simulink subsystem "trajectory_generation_ref_subsys_cont"  (R2023b)
settings: Solver=VariableStepAuto  StartTime=0.0  StopTime=10.0  RelTol=1e-3
values from neighbouring files (symbols this model uses):
  H_0_init = [7.85046229342e-17 1 0 0 1 -7.85046229342e-17 0 0 0 0 -1 0 ... (16 elements, 4x4)]    [matlab.mat]    (also in parameters.m = hom_transform_endeffector(q_0, param_robot))
  param_traj_allg =     [matlab.mat]
  xe0 = [0.392090710168 0.392090710168 0.5211 0 0.707106781187 0.707106781187 0]    [matlab.mat]    (also in parameters.m = temp)
  xeT = [0.392090710168 0.392090710168 0.5211 0 0.382683432365 0.923879532511 0]    [matlab.mat]    (also in parameters.m = xe0)
settings Model: Creator=emu  LastModifiedBy=emu

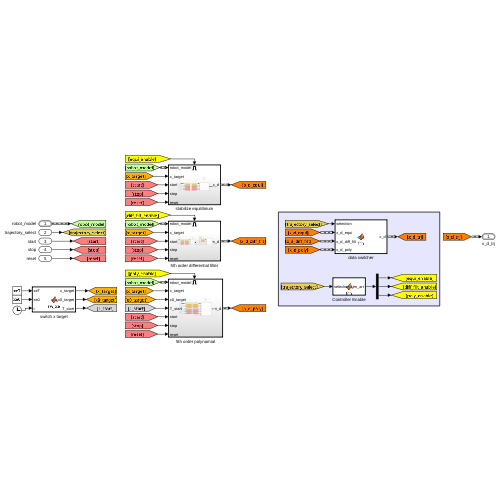
[thumbnail: Simulink's stored preview of the top-level diagram]
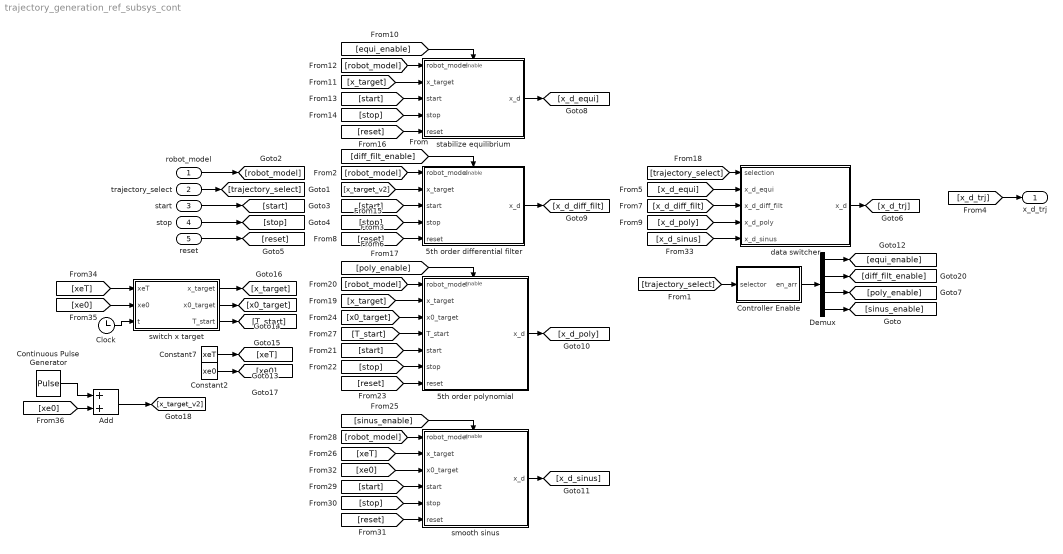
== system trajectory_generation_ref_subsys_cont ==
  robot_model : Inport  OutDataTypeStr=Bus: robot_model
  trajectory_select : Inport  Port=2
  start : Inport  Port=3
  stop : Inport  Port=4
  reset : Inport  Port=5
  5th order differential filter : Subsystem
  5th order polynomial : Subsystem
  Add : Sum
  Clock : Clock
  Constant2 : Constant  Value=xe0
  Constant7 : Constant  Value=xeT
  Continuous Pulse Generator : DiscretePulseGenerator  PulseType=Time based  Amplitude=xeT-xe0  Period=param_traj_allg.T_switch*2  PulseWidth=50
  Controller Enable : MATLAB Function  TreatAsAtomicUnit=on
  Demux : Demux
  data switcher : MATLAB Function  TreatAsAtomicUnit=on
  smooth sinus : Subsystem
  stabilize equilibrium : Subsystem
  switch x target : MATLAB Function  TreatAsAtomicUnit=on
  x_d_trj : Outport  OutDataTypeStr=Bus: x_d
  wires:
  [reset] -> 5th order differential filter/5(reset)
  [x_d_equi] -> data switcher/2(x_d_equi)
  [poly_enable] -> 5th order polynomial/Enable
  [x_target] -> stabilize equilibrium/2(x_target)
  [robot_model] -> 5th order differential filter/1(robot_model)
  Clock/1 -> switch x target/3(t)
  [xe0] -> switch x target/2(xe0)
  stop/1 -> [stop]
  Demux/2 -> [diff_filt_enable]
  switch x target/2(x0_target) -> [x0_target]
  start/1 -> [start]
  Demux/3 -> [poly_enable]
  [diff_filt_enable] -> 5th order differential filter/Enable
  [reset] -> stabilize equilibrium/5(reset)
  reset/1 -> [reset]
  [stop] -> 5th order polynomial/6(stop)
  5th order polynomial/1(x_d) -> [x_d_poly]
  [stop] -> 5th order differential filter/4(stop)
  [x_d_poly] -> data switcher/4(x_d_poly)
  data switcher/1(x_d) -> [x_d_trj]
  [T_start] -> 5th order polynomial/4(T_start)
  [x_d_trj] -> x_d_trj/1
  [x_target_v2] -> 5th order differential filter/2(x_target)
  [x_target] -> 5th order polynomial/2(x_target)
  switch x target/3(T_start) -> [T_start]
  [robot_model] -> 5th order polynomial/1(robot_model)
  robot_model/1 -> [robot_model]
  trajectory_select/1 -> [trajectory_select]
  [x0_target] -> 5th order polynomial/3(x0_target)
  [trajectory_select] -> Controller Enable/1(selector)
  [stop] -> stabilize equilibrium/4(stop)
  [start] -> stabilize equilibrium/3(start)
  stabilize equilibrium/1(x_d) -> [x_d_equi]
  5th order differential filter/1(x_d) -> [x_d_diff_filt]
  [robot_model] -> stabilize equilibrium/1(robot_model)
  [reset] -> 5th order polynomial/7(reset)
  [x_d_diff_filt] -> data switcher/3(x_d_diff_filt)
  switch x target/1(x_target) -> [x_target]
  Controller Enable/1(en_arr) -> Demux/1
  [start] -> 5th order polynomial/5(start)
  [xeT] -> switch x target/1(xeT)
  [equi_enable] -> stabilize equilibrium/Enable
  Demux/1 -> [equi_enable]
  [trajectory_select] -> data switcher/1(selection)
  [start] -> 5th order differential filter/3(start)
  [start] -> smooth sinus/4(start)
  [reset] -> smooth sinus/6(reset)
  [xe0] -> smooth sinus/3(x0_target)
  [robot_model] -> smooth sinus/1(robot_model)
  [xeT] -> smooth sinus/2(x_target)
  smooth sinus/1(x_d) -> [x_d_sinus]
  [stop] -> smooth sinus/5(stop)
  [sinus_enable] -> smooth sinus/Enable
  Demux/4 -> [sinus_enable]
  [x_d_sinus] -> data switcher/5(x_d_sinus)
  Constant7/1 -> [xeT]
  Constant2/1 -> [xe0]
  Continuous Pulse Generator/1 -> Add/1
  [xe0] -> Add/2
  Add/1 -> [x_target_v2]

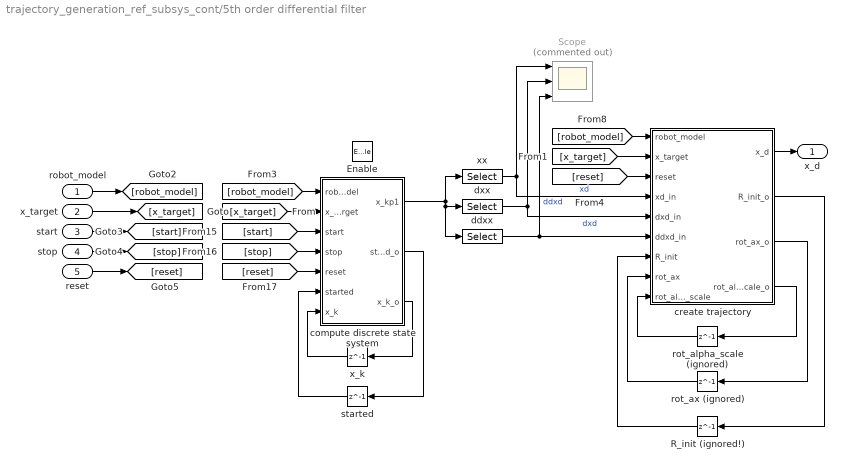
== system trajectory_generation_ref_subsys_cont/5th order differential filter ==
  robot_model : Inport
  x_target : Inport  Port=2
  start : Inport  Port=3
  stop : Inport  Port=4
  reset : Inport  Port=5
  Enable : EnablePort
  R_init (ignored!) : Delay  DelayLength=1  InitialCondition=eye(3)
  Scope : Scope  Commented=on  NumInputPorts=3
  compute discrete state system : MATLAB Function  TreatAsAtomicUnit=on
  create trajectory : MATLAB Function  TreatAsAtomicUnit=on
  ddxx : Selector  InputPortWidth=24  IndexOptions=Index vector (dialog)  Indices=selector_index3  OutputSizes=1
  dxx : Selector  InputPortWidth=24  IndexOptions=Index vector (dialog)  Indices=selector_index2  OutputSizes=1
  rot_alpha_scale (ignored) : Delay  DelayLength=1  InitialCondition=0
  rot_ax (ignored) : Delay  DelayLength=1  InitialCondition=[1;0;0]
  started : Delay  DelayLength=1
  x_k : Delay  DelayLength=1  InitialCondition=[reshape([H_0_init(1:3,4) zeros(3,5)]', 6*3,1)]
  xx : Selector  InputPortWidth=24  IndexOptions=Index vector (dialog)  Indices=selector_index1  OutputSizes=1
  x_d : Outport  OutDataTypeStr=Bus: x_d
  wires:
  R_init (ignored!)/1 -> create trajectory/7(R_init)
  rot_ax (ignored)/1 -> create trajectory/8(rot_ax)
  rot_alpha_scale (ignored)/1 -> create trajectory/9(rot_alpha_scale)
  create trajectory/2(R_init_o) -> R_init (ignored!)/1
  create trajectory/3(rot_ax_o) -> rot_ax (ignored)/1
  create trajectory/4(rot_alpha_scale_o) -> rot_alpha_scale (ignored)/1
  started/1 -> compute discrete state system/6(started)
  x_k/1 -> compute discrete state system/7(x_k)
  compute discrete state system/3(x_k_o) -> x_k/1
  compute discrete state system/2(started_o) -> started/1
  [x_target] -> compute discrete state system/2(x_target)
  [x_target] -> create trajectory/2(x_target)
  x_target/1 -> [x_target]
  ddxx/1 -> create trajectory/6(ddxd_in), Scope/3  "ddxd"
  [start] -> compute discrete state system/3(start)
  xx/1 -> Scope/1, create trajectory/4(xd_in)  "xd"
  [robot_model] -> compute discrete state system/1(robot_model)
  [stop] -> compute discrete state system/4(stop)
  create trajectory/1(x_d) -> x_d/1
  dxx/1 -> Scope/2, create trajectory/5(dxd_in)  "dxd"
  compute discrete state system/1(x_kp1) -> xx/1, dxx/1, ddxx/1
  [reset] -> compute discrete state system/5(reset)
  robot_model/1 -> [robot_model]
  start/1 -> [start]
  reset/1 -> [reset]
  [reset] -> create trajectory/3(reset)
  stop/1 -> [stop]
  [robot_model] -> create trajectory/1(robot_model)

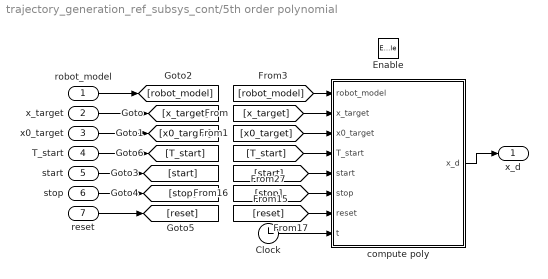
== system trajectory_generation_ref_subsys_cont/5th order polynomial ==
  robot_model : Inport
  x_target : Inport  Port=2
  x0_target : Inport  Port=3
  T_start : Inport  Port=4
  start : Inport  Port=5
  stop : Inport  Port=6
  reset : Inport  Port=7
  Enable : EnablePort
  Clock : Clock
  compute poly : MATLAB Function  TreatAsAtomicUnit=on
  x_d : Outport  OutDataTypeStr=Bus: x_d
  wires:
  [T_start] -> compute poly/4(T_start)
  T_start/1 -> [T_start]
  [x0_target] -> compute poly/3(x0_target)
  x0_target/1 -> [x0_target]
  Clock/1 -> compute poly/8(t)
  [start] -> compute poly/5(start)
  [stop] -> compute poly/6(stop)
  compute poly/1(x_d) -> x_d/1
  [reset] -> compute poly/7(reset)
  robot_model/1 -> [robot_model]
  start/1 -> [start]
  reset/1 -> [reset]
  stop/1 -> [stop]
  x_target/1 -> [x_target]
  [x_target] -> compute poly/2(x_target)
  [robot_model] -> compute poly/1(robot_model)

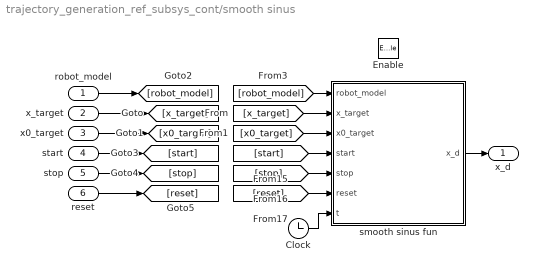
== system trajectory_generation_ref_subsys_cont/smooth sinus ==
  robot_model : Inport
  x_target : Inport  Port=2
  x0_target : Inport  Port=3
  start : Inport  Port=4
  stop : Inport  Port=5
  reset : Inport  Port=6
  Enable : EnablePort
  Clock : Clock
  smooth sinus fun : MATLAB Function  TreatAsAtomicUnit=on
  x_d : Outport  OutDataTypeStr=Bus: x_d
  wires:
  [robot_model] -> smooth sinus fun/1(robot_model)
  [x_target] -> smooth sinus fun/2(x_target)
  x_target/1 -> [x_target]
  stop/1 -> [stop]
  reset/1 -> [reset]
  start/1 -> [start]
  robot_model/1 -> [robot_model]
  [reset] -> smooth sinus fun/6(reset)
  smooth sinus fun/1(x_d) -> x_d/1
  [stop] -> smooth sinus fun/5(stop)
  [start] -> smooth sinus fun/4(start)
  Clock/1 -> smooth sinus fun/7(t)
  x0_target/1 -> [x0_target]
  [x0_target] -> smooth sinus fun/3(x0_target)

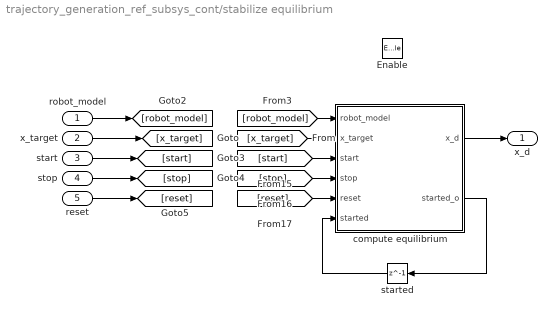
== system trajectory_generation_ref_subsys_cont/stabilize equilibrium ==
  robot_model : Inport
  x_target : Inport  Port=2
  start : Inport  Port=3
  stop : Inport  Port=4
  reset : Inport  Port=5
  Enable : EnablePort
  compute equilibrium : MATLAB Function  TreatAsAtomicUnit=on
  started : Delay  DelayLength=1
  x_d : Outport  OutDataTypeStr=Bus: x_d
  wires:
  compute equilibrium/2(started_o) -> started/1
  started/1 -> compute equilibrium/6(started)
  [robot_model] -> compute equilibrium/1(robot_model)
  [x_target] -> compute equilibrium/2(x_target)
  x_target/1 -> [x_target]
  stop/1 -> [stop]
  reset/1 -> [reset]
  start/1 -> [start]
  robot_model/1 -> [robot_model]
  [reset] -> compute equilibrium/5(reset)
  compute equilibrium/1(x_d) -> x_d/1
  [stop] -> compute equilibrium/4(stop)
  [start] -> compute equilibrium/3(start)

== matlab function trajectory_generation_ref_subsys_cont/switch x target ==
  data: x_target output; x0_target output; xeT input; xe0 input; t input; param_vis parameter; T_start output
function [x_target, x0_target, T_start]= sw_xe(xeT, xe0, t, param_vis)

if(t < param_vis.T/2)
    x_target = xeT;
    x0_target = xe0;
    flag = 0;
else
    x_target = xe0;
    x0_target = xeT;
    flag = 1;
end

if(flag == 0)
    T_start = 0;
else
    T_start = param_vis.T/2;
end

== matlab function trajectory_generation_ref_subsys_cont/smooth sinus/smooth sinus fun ==
  settings: sampleTime=param_global.Ta
  data: robot_model input Bus: robot_model; x_target input; x0_target input; start input; stop input; reset input; t input; x_d output Bus: x_d; param_traj_sin_poly parameter
function x_d  = ss_z(robot_model, x_target, x0_target, start, stop, reset, t, param_traj_sin_poly)

persistent started;

if(reset == 1 || isempty(started))
    started = false;
end

if(start == 1 && stop == 0 && ~started)
    started = true;
end

if(stop == 1)
    started = false;
end

if(started)
    T = param_traj_sin_poly.T;
    omega = param_traj_sin_poly.omega;
    phi = param_traj_sin_poly.phi;
    if(t > T)
        s =    1;
        s_p =  0;
        s_pp = 0;
    else
        [s, s_p, s_pp] = trajectory_poly(t, 0, 1, T);
    end
    xT = x_target(1);
    x0 = x0_target(1);

    a = (xT - x0)/2; % width of sinus movement

    sin_t = a*sin(omega*t - phi);
    cos_t = a*cos(omega*t - phi);

    %p_d = x0 + a*sin(omega*t)*s;
    %p_d_p = a*omega*cos(omega*t)*s + a*sin(omega*t)*s_p;
    %p_d_pp = -omega*a*sin(omega*t)*s + 2*omega*cos(omega*t)*s_p + a*sin(omega*t) * s_pp;
    x_ref = x0 + (a + sin_t) * s;
    x_ref_p =    cos_t * omega * s   + sin_t * s_p;
    x_ref_pp =  -sin_t * omega^2 * s + cos_t * s_p * omega * 2 + sin_t * s_pp;

    x_d.p_d = [x_ref; x_target(2:3)];
    x_d.p_d_p = [x_ref_p; x_target(2:3)];
    x_d.p_d_pp = [x_ref_pp; x_target(2:3)];
    
    x_d.q_d = zeros(4,1);
    x_d.omega_d   = zeros(3,1);
    x_d.omega_d_p = zeros(3,1);
else
    H = robot_model.H;
    p_e = H(1:3, 4);

    x_d.p_d = p_e;
    x_d.p_d_p =  zeros(3,1);
    x_d.p_d_pp = zeros(3,1);
    x_d.q_d = zeros(4,1);
    x_d.omega_d   = zeros(3,1);
    x_d.omega_d_p = zeros(3,1);
end

== matlab function trajectory_generation_ref_subsys_cont/5th order differential filter/compute discrete state system ==
  settings: sampleTime=param_global.Ta
  data: robot_model input Bus: robot_model; x_target input; start input; stop input; reset input; started input; x_k input; x_kp1 output; param_traj_filter parameter; started_o output; x_k_o output
function [x_kp1, started_o, x_k_o]  = ss_z(robot_model, x_target, start, stop, reset, started, x_k, param_traj_filter)

if(reset == 1)
    H = robot_model.H;
    yt_init = H(1:3, 4);
    %x_target = eval_path_t(theta, 1, path_param);
    %x;d/dt x;d^2/dt^2 x; y;d/dt y;d^2/dt^2 y; z;d/dt z;d^2/dt^2 z; alpha;d/dt alpha;d^2/dt^2 alpha
    x_0 = [yt_init(1);0;0;0;0;0; yt_init(2);0;0;0;0;0; yt_init(3);0;0;0;0;0; 0;0;0;0;0;0];
    x_k = x_0;
    started = false;
end

if(start == 1 && stop == 0 && ~started)
    started = true;
end

if(stop == 1)
    started = false;
end

if(started)
    Phi = param_traj_filter.Phi;
    Gamma = param_traj_filter.Gamma;
    alpha_T = 1; % die idee ist, dass alpha \in [0,1] ist, da man die Drehung normiert durchführt.
    x_kp1 = Phi*x_k + Gamma*[x_target(1:3);alpha_T];
else
    x_kp1 = x_k;
end
x_k_o = x_kp1;
started_o = started;

== matlab function trajectory_generation_ref_subsys_cont/5th order differential filter/create trajectory ==
  settings: sampleTime=param_global.Ta
  data: robot_model input Bus: robot_model; x_target input; reset input; xd_in input; dxd_in input; ddxd_in input; x_d output Bus: x_d; R_init input; rot_ax input; rot_alpha_scale input; R_init_o output; rot_ax_o output; rot_alpha_scale_o output
function [x_d, R_init_o, rot_ax_o, rot_alpha_scale_o]  = trajectory(robot_model, x_target, reset, xd_in, dxd_in, ddxd_in, R_init, rot_ax, rot_alpha_scale)

if(reset)
    H = robot_model.H;
    R_init = H(1:3, 1:3);

    %R_target = eval_path_r(theta,1,path_param);
    R_target = eul2rotm(x_target(4:6)', "ZYZ");
    RR = R_init'*R_target;
    rot_quat = rotation2quaternion(RR);
    rot_rho = rot_quat(1);
    rot_alpha_scale = 2*acos(rot_rho);
    rot_ax = rot_quat(2:4)/sin(rot_alpha_scale/2);

    % rot_alpha_scale gibt den winkel an, den man ausgehend von der
    % Orientierung Rt um die Rotationsachse rot_ax drehen müsste, bis man
    % in die Zielorientierung ReT_in kommt. Da in xd_in(4) der Winkel alpha
    % steht für den man die Ableitungen in dxd_in(4) und ddxd_in(4) über
    % die Sollwertfilter berechnet hat und dieser Winkel im range 0 bis 1
    % ist, benötigt man rot_alpha_scale damit die Drehung bei alpha=1 auch
    % tatsächlich durchgeführt wurde.
end

x_d.p_d =    xd_in(1:3);
x_d.p_d_p =  dxd_in(1:3);
x_d.p_d_pp = ddxd_in(1:3);

alpha =   xd_in(4);
alpha_p =  dxd_in(4);
alpha_pp = ddxd_in(4);

skew_ew = skew(rot_ax);
R_act = R_init*(eye(3) + sin(rot_alpha_scale*alpha)*skew_ew + (1-cos(rot_alpha_scale*alpha))*skew_ew^2);

x_d.q_d = rotation2quaternion(R_act);
x_d.omega_d   = alpha_p*rot_ax;
x_d.omega_d_p = alpha_pp*rot_ax;

R_init_o = R_init;
rot_ax_o = rot_ax;
rot_alpha_scale_o = rot_alpha_scale;

== matlab function trajectory_generation_ref_subsys_cont/5th order polynomial/compute poly ==
  settings: sampleTime=param_global.Ta
  data: robot_model input Bus: robot_model; x_target input; x0_target input; T_start input; start input; stop input; reset input; t input; x_d output Bus: x_d; param_traj_poly parameter
function x_d  = ss_z(robot_model, x_target, x0_target, T_start, start, stop, reset, t, param_traj_poly)

persistent started;
persistent R_init;
persistent rot_ax;
persistent rot_alpha_scale;

if(isempty(rot_ax) || reset)
    H = robot_model.H;
    R_init = H(1:3, 1:3);

    %R_target = eval_path_r(theta,1,path_param);
    R_target = eul2rotm(x_target(4:6)', "ZYZ");
    RR = R_init'*R_target;
    rot_quat = rotation2quaternion(RR);
    rot_rho = rot_quat(1);
    rot_alpha_scale = 2*acos(rot_rho);
    rot_ax = rot_quat(2:4)/sin(rot_alpha_scale/2);

    % rot_alpha_scale gibt den winkel an, den man ausgehend von der
    % Orientierung Rt um die Rotationsachse rot_ax drehen müsste, bis man
    % in die Zielorientierung ReT_in kommt. Da in xd_in(4) der Winkel alpha
    % steht für den man die Ableitungen in dxd_in(4) und ddxd_in(4) über
    % die Sollwertfilter berechnet hat und dieser Winkel im range 0 bis 1
    % ist, benötigt man rot_alpha_scale damit die Drehung bei alpha=1 auch
    % tatsächlich durchgeführt wurde.
    started = false;
end

if(start == 1 && stop == 0 && ~started)
    started = true;
end

if(stop == 1)
    started = false;
end

if(started)
    T = param_traj_poly.T;
    if(t-T_start > T)
        p_d =    [x_target(1:3); 1];
        p_d_p =  [zeros(3,1); 1];
        p_d_pp = [zeros(3,1); 1];
    else
        yT = [x_target(1:3); 1]; % poly contains [x,y,z,alpha]
        y0 = [x0_target(1:3); 0];
        [p_d, p_d_p, p_d_pp] = trajectory_poly(t-T_start, y0, yT, T);
    end
    x_d.p_d = p_d(1:3);
    x_d.p_d_p =  p_d_p(1:3);
    x_d.p_d_pp = p_d_pp(1:3);

    alpha = p_d(4);
    alpha_p = p_d_p(4);
    alpha_pp = p_d_pp(4);
    skew_ew = skew(rot_ax);
    R_act = R_init*(eye(3) + sin(rot_alpha_scale*alpha)*skew_ew + (1-cos(rot_alpha_scale*alpha))*skew_ew^2);
    
    x_d.q_d = rotation2quaternion(R_act);
    x_d.omega_d   = alpha_p*rot_ax;
    x_d.omega_d_p = alpha_pp*rot_ax;
else
    H = robot_model.H;
    p_e = H(1:3, 4);
    R_e = H(1:3,1:3);

    x_d.p_d = p_e(1:3);
    x_d.p_d_p =  zeros(3,1);
    x_d.p_d_pp = zeros(3,1);
    x_d.q_d = rotation2quaternion(R_e);
    x_d.omega_d   = zeros(3,1);
    x_d.omega_d_p = zeros(3,1);
end

== matlab function trajectory_generation_ref_subsys_cont/Controller Enable ==
  settings: sampleTime=param_global.Ta
  data: en_arr output; selector input uint32
function en_arr  = fcn(selector)
    % Wichtig: selector \in [1,max(selector)]
    % Es wird ein bool array ausgegeben, welches nur den index 1 setzt, der
    % mit selector übereinstimmt. Achtung: Size von "en_arr" muss
    % entsprechend der Ausgänge unter "Edit Data" manuell angegeben werden.
    % Beispiel: 4 Inputs, max(selector)=4, Size = [1 4]
    % z. B. selector = 2
    % 1:4 == selector liefert [0 1 0 0]
    en_arr = (1:4 == selector)';
end

== matlab function trajectory_generation_ref_subsys_cont/data switcher ==
  settings: sampleTime=param_global.Ta
  data: selection input; x_d_equi input Bus: x_d; x_d_diff_filt input Bus: x_d; x_d output Bus: x_d; x_d_poly input Bus: x_d; x_d_sinus input Bus: x_d
function x_d   = fcn(selection, x_d_equi, x_d_diff_filt, x_d_poly, x_d_sinus)

if(selection == 1)
    x_d = x_d_equi;
elseif(selection == 2)
    x_d = x_d_diff_filt;
elseif(selection == 3)
    x_d = x_d_poly;
else
    x_d = x_d_sinus;
end

== matlab function trajectory_generation_ref_subsys_cont/stabilize equilibrium/compute equilibrium ==
  settings: sampleTime=param_global.Ta
  data: robot_model input Bus: robot_model; x_target input; start input; stop input; reset input; x_d output Bus: x_d; started input; started_o output
function [x_d, started_o]  = ss_z(robot_model, x_target, start, stop, reset, started)

if(reset == 1 || stop == 1)
    started = false;
end

if(start == 1 && stop == 0 && ~started)
    started = true;
end

if(started)
    x_d.p_d = x_target(1:3);
    x_d.p_d_p =  zeros(3,1);
    x_d.p_d_pp = zeros(3,1);
    x_d.q_d = rotation2quaternion(eul2rotm(x_target(4:6)', "ZYZ"));
    x_d.omega_d   = zeros(3,1);
    x_d.omega_d_p = zeros(3,1);
else
    H = robot_model.H;
    p_e = H(1:3, 4);
    R_e = H(1:3,1:3);

    x_d.p_d = p_e(1:3);
    x_d.p_d_p =  zeros(3,1);
    x_d.p_d_pp = zeros(3,1);
    x_d.q_d = rotation2quaternion(R_e);
    x_d.omega_d   = zeros(3,1);
    x_d.omega_d_p = zeros(3,1);
end
